simulink model "Engine_Model_HIL"  (R2016b)
settings: Solver=FixedStepDiscrete  StartTime=0.0  StopTime=inf  FixedStep=EngMdl.tiSimnTiStep_C  RelTol=1e-3  EnableMultiTasking=on
undefined symbols (not defined in the file or in its folder): EngMdl
libraries: gtlink2017rt x1, simulink x1
(part 1 of 2)
settings Model: Creator=m01wolf  LastModifiedBy=bunver
settings DataIOCC: SaveFormat=StructureWithTime  SaveOutput=off  DSMLogging=off  VisualizeSimOutput=off  SaveTime=off  StateSaveName=Results  SignalLoggingName=Results
settings OptimizationCC: BlockReduction=off  ConditionallyExecuteInputs=off  LifeSpan=inf
settings DebuggingCC: AllowSymbolicDim=off  SFUnexpectedBacktrackingDiag=warning  SFNoUnconditionalDefaultTransitionDiag=warning  SFExecutionAtInitializationDiag=none
settings ModelReferenceCC: ModelReferenceNumInstancesAllowed=Single  PropagateSignalLabelsOutOfModel=off
settings GRTTargetCC: TargetLangStandard=C89/C90 (ANSI)
settings ConfigComp: CovMetricSettings=dw  CovHtmlReporting=on  CovSaveCumulativeToWorkspaceVar=on  CovSaveSingleToWorkspaceVar=on  CovExternalEMLEnable=off

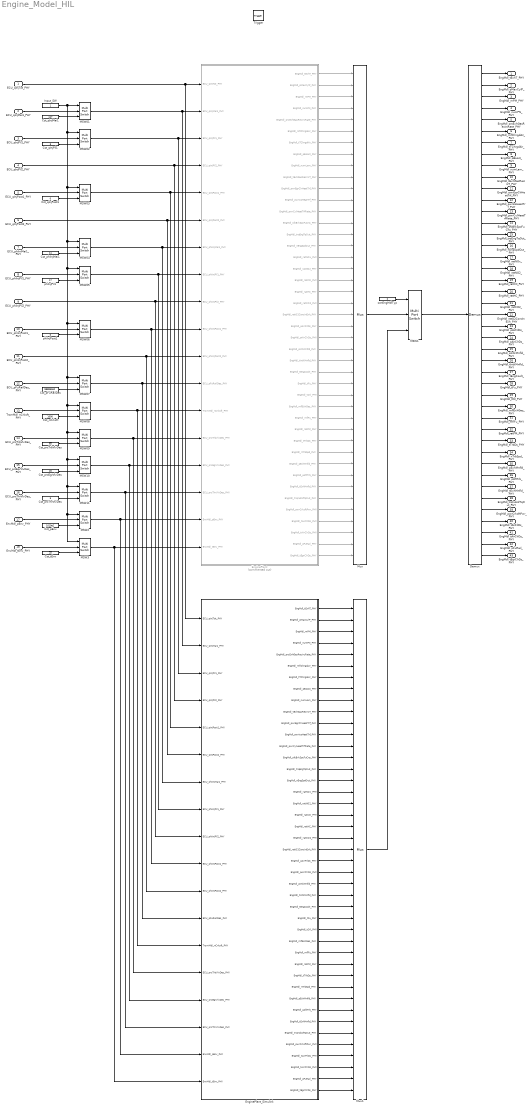
== system Engine_Model_HIL ==
  ECU_qInjTot_PHY : Inport
  ECU_qInjMai1_PHY : Inport  Port=2
  ECU_qInjPil1_PHY : Inport  Port=3
  ECU_qInjPil2_PHY : Inport  Port=4
  ECU_qInjPost1_PHY : Inport  Port=5
  ECU_qInjPost2_PHY : Inport  Port=6
  ECU_phiInjMai1_PHY : Inport  Port=7
  ECU_phiInjPil1_PHY : Inport  Port=8
  ECU_phiInjPil2_PHY : Inport  Port=9
  ECU_phiInjPost1_PHY : Inport  Port=10
  ECU_phiInjPost2_PHY : Inport  Port=11
  ECU_pFuRailDes_PHY : Inport  Port=12
  TrsmMdl_nCrksft_PHY : Inport  Port=13
  ECU_prcTrbVlvDes_PHY : Inport  Port=14
  ECU_prcEgrVlvDes_PHY : Inport  Port=15
  ECU_prcThrVlvDes_PHY : Inport  Port=16
  EnvMdl_pEnv_PHY : Inport  Port=17
  EnvMdl_tEnv_PHY : Inport  Port=18
  Trigger : TriggerPort  TriggerType=function-call  VariantControl=Variant  SampleTime=EngMdl.tiSimnTiStep_C  PortDimensions=1
  Cst_nCrksft : Constant  Value=1000  SampleTime=-1
  Cst_pEnv : Constant  Value=1010e2  SampleTime=-1
  Cst_pFuRailDes : Constant  Value=988853e2  SampleTime=-1
  Cst_phiInjMai1 : Constant  Value=11  SampleTime=-1
  Cst_prcEgrVlvDes : Constant  Value=20  SampleTime=-1
  Cst_prcThrVlvDes : Constant  Value=5  SampleTime=-1
  Cst_prcTrbVlvDes : Constant  Value=65  SampleTime=-1
  Cst_qInjMai1 : Constant  Value=147  SampleTime=-1
  Cst_qInjPil1 : Constant  Value=3  SampleTime=-1
  Cst_qInjPost1 : Constant  Value=0  SampleTime=-1
  Cst_tEnv : Constant  Value=25  SampleTime=-1
  Demux : Demux  Outputs=43
  EnginePlant : Subsystem  Commented=on
  EnginePlant_Simulink : Subsystem
  Input_SW : Constant  SampleTime=-1
  MSW01 : MultiPortSwitch  Inputs=2
  MSW02 : MultiPortSwitch  Inputs=2
  MSW03 : MultiPortSwitch  Inputs=2
  MSW04 : MultiPortSwitch  Inputs=2
  MSW05 : MultiPortSwitch  Inputs=2
  MSW06 : MultiPortSwitch  Inputs=2
  MSW07 : MultiPortSwitch  Inputs=2
  MSW08 : MultiPortSwitch  Inputs=2
  MSW09 : MultiPortSwitch  Inputs=2
  MSW{1..3,10..11} (5 alike) : MultiPortSwitch  Inputs=2
  Mux : Mux  Inputs=43
  Mux1 : Mux  Inputs=43
  phiInjPil1 : Constant  Value=17  SampleTime=-1
  phiInjPost1 : Constant  Value=0  SampleTime=-1
  swtEngMdlTyp : Constant  Value=2  SampleTime=-1
  EngMdl_tExhT_PHY : Outport  OutMin=-21  OutMax=2147
  EngMdl_pMaxCylP_PHY : Outport  Port=2  OutMin=-21  OutMax=2147
  EngMdl_mPM_PHY : Outport  Port=3  OutMin=-21  OutMax=2147
  EngMdl_numPN_PHY : Outport  Port=4  OutMin=-21  OutMax=200000000
  EngMdl_prcExhGasRecircRate_PHY : Outport  Port=5  OutMin=-21  OutMax=200
  EngMdl_mflChrgdAir_PHY : Outport  Port=6  OutMin=-21  OutMax=2147487
  EngMdl_tTChrgdAir_PHY : Outport  Port=7  OutMin=-50  OutMax=257
  EngMdl_pBoost_PHY : Outport  Port=8  OutMin=-1  OutMax=12
  EngMdl_numLam_PHY : Outport  Port=9  OutMin=-1  OutMax=15
  EngMdl_tExhGasRecircT_PHY : Outport  Port=10  OutMin=-21  OutMax=2000
  EngMdl_pwrEgrClrHeatTrf_PHY : Outport  Port=11  OutMin=-32768  OutMax=32767
  EngMdl_pwrIcoHeatTrf_PHY : Outport  Port=12  OutMin=-32768  OutMax=32767
  EngMdl_pwrCylHeatTrfRate_PHY : Outport  Port=13  OutMin=-2147483648  OutMax=2147483647
  EngMdl_sfcBrkSpcFuCns_PHY : Outport  Port=14  OutMin=-214  OutMax=2147
  EngMdl_trqEngTqOut_PHY : Outport  Port=15  OutMin=-21470  OutMax=214748
  EngMdl_nEngSpdOut_PHY : Outport  Port=16  OutMin=-21470  OutMax=21474
  EngMdl_ratNOx_PHY : Outport  Port=17  OutMin=-21  OutMax=214700
  EngMdl_ratNO2_PHY : Outport  Port=18  OutMin=-21  OutMax=214700
  EngMdl_ratCO_PHY : Outport  Port=19  OutMin=-21  OutMax=214700
  EngMdl_ratHC_PHY : Outport  Port=20  OutMin=-21  OutMax=214700
  EngMdl_ratCO2_PHY : Outport  Port=21  OutMin=-21  OutMax=20000000
  EngMdl_ratO2ConcInExh_PHY : Outport  Port=22  OutMin=-2147483648  OutMax=2147483647
  EngMdl_pAirFilDs_PHY : Outport  Port=23  OutMin=0  OutMax=1000000
  EngMdl_pAirClrDs_PHY : Outport  Port=24  OutMin=0  OutMax=1000000
  EngMdl_pIntkMnfld_PHY : Outport  Port=25  OutMin=0  OutMax=1000000
  EngMdl_tIntkMnfld_PHY : Outport  Port=26  OutMin=-250  OutMax=1000
  EngMdl_tEngCoolt_PHY : Outport  Port=27  OutMin=-250  OutMax=1000
  EngMdl_tFu_PHY : Outport  Port=28  OutMin=-250  OutMax=1000
  EngMdl_tOil_PHY : Outport  Port=29  OutMin=-250  OutMax=1000
  EngMdl_mflExhGas_PHY : Outport  Port=30
  EngMdl_mflFu_PHY : Outport  Port=31
  EngMdl_ratPM_PHY : Outport  Port=32
  EngMdl_tTrbDs_PHY : Outport  Port=33
  EngMdl_nTrbSpd_PHY : Outport  Port=34
  EngMdl_pExhMnfld_PHY : Outport  Port=35
  EngMdl_pAftTrb_PHY : Outport  Port=36
  EngMdl_tExhMnfld_PHY : Outport  Port=37
  EngMdl_trqIndcdTqOut_PHY : Outport  Port=38
  EngMdl_pwrCrksftPwr_PHY : Outport  Port=39
  EngMdl_tAirFilDs_PHY : Outport  Port=40
  EngMdl_tAirClrDs_PHY : Outport  Port=41
  EngMdl_pFuRail_PHY : Outport  Port=42
  EngMdl_tEgrClrDs_PHY : Outport  Port=43
  wires:
  ECU_qInjTot_PHY/1 -> EnginePlant_Simulink/1(ECU_qInjTot_PHY), EnginePlant/1(ECU_qInjTot_PHY)
  ECU_qInjPil2_PHY/1 -> EnginePlant/4(ECU_qInjPil2_PHY), EnginePlant_Simulink/4(ECU_qInjPil2_PHY)
  ECU_qInjPost2_PHY/1 -> EnginePlant/6(ECU_qInjPost2_PHY), EnginePlant_Simulink/6(ECU_qInjPost2_PHY)
  ECU_phiInjPil2_PHY/1 -> EnginePlant/9(ECU_phiInjPil2_PHY), EnginePlant_Simulink/9(ECU_phiInjPil2_PHY)
  ECU_phiInjPost2_PHY/1 -> EnginePlant/11(ECU_phiInjPost2_PHY), EnginePlant_Simulink/11(ECU_phiInjPost2_PHY)
  Cst_qInjMai1/1 -> MSW01/3
  Cst_qInjPil1/1 -> MSW02/3
  phiInjPil1/1 -> MSW05/3
  Cst_phiInjMai1/1 -> MSW04/3
  Cst_pFuRailDes/1 -> MSW07/3
  Cst_nCrksft/1 -> MSW08/3
  Cst_prcTrbVlvDes/1 -> MSW09/3
  Cst_prcThrVlvDes/1 -> MSW11/3
  Cst_prcEgrVlvDes/1 -> MSW10/3
  MSW01/1 -> EnginePlant/2(ECU_qInjMai1_PHY), EnginePlant_Simulink/2(ECU_qInjMai1_PHY)
  MSW02/1 -> EnginePlant/3(ECU_qInjPil1_PHY), EnginePlant_Simulink/3(ECU_qInjPil1_PHY)
  ECU_qInjPil1_PHY/1 -> MSW02/2
  ECU_qInjMai1_PHY/1 -> MSW01/2
  MSW04/1 -> EnginePlant/7(ECU_phiInjMai1_PHY), EnginePlant_Simulink/7(ECU_phiInjMai1_PHY)
  ECU_phiInjMai1_PHY/1 -> MSW04/2
  MSW05/1 -> EnginePlant/8(ECU_phiInjPil1_PHY), EnginePlant_Simulink/8(ECU_phiInjPil1_PHY)
  ECU_phiInjPil1_PHY/1 -> MSW05/2
  MSW07/1 -> EnginePlant/12(ECU_pFuRailDes_PHY), EnginePlant_Simulink/12(ECU_pFuRailDes_PHY)
  ECU_pFuRailDes_PHY/1 -> MSW07/2
  MSW08/1 -> EnginePlant/13(TrsmMdl_nCrksft_PHY), EnginePlant_Simulink/13(TrsmMdl_nCrksft_PHY)
  TrsmMdl_nCrksft_PHY/1 -> MSW08/2
  MSW09/1 -> EnginePlant/14(ECU_prcTrbVlvDes_PHY), EnginePlant_Simulink/14(ECU_prcTrbVlvDes_PHY)
  ECU_prcTrbVlvDes_PHY/1 -> MSW09/2
  ECU_prcEgrVlvDes_PHY/1 -> MSW10/2
  MSW10/1 -> EnginePlant/15(ECU_prcEgrVlvDes_PHY), EnginePlant_Simulink/15(ECU_prcEgrVlvDes_PHY)
  MSW11/1 -> EnginePlant/16(ECU_prcThrVlvDes_PHY), EnginePlant_Simulink/16(ECU_prcThrVlvDes_PHY)
  ECU_prcThrVlvDes_PHY/1 -> MSW11/2
  Input_SW/1 -> MSW02/1, MSW03/1, MSW04/1, MSW05/1, MSW06/1, MSW07/1, MSW08/1, MSW09/1, MSW10/1, MSW2/1, MSW3/1, MSW11/1, MSW01/1
  phiInjPost1/1 -> MSW06/3
  MSW06/1 -> EnginePlant/10(ECU_phiInjPost1_PHY), EnginePlant_Simulink/10(ECU_phiInjPost1_PHY)
  ECU_phiInjPost1_PHY/1 -> MSW06/2
  Cst_qInjPost1/1 -> MSW03/3
  MSW03/1 -> EnginePlant/5(ECU_qInjPost1_PHY), EnginePlant_Simulink/5(ECU_qInjPost1_PHY)
  ECU_qInjPost1_PHY/1 -> MSW03/2
  EnginePlant_Simulink/37(EngMdl_tExhMnfld_PHY) -> Mux1/37
  EnginePlant_Simulink/7(EngMdl_tTChrgdAir_PHY) -> Mux1/7
  EnginePlant_Simulink/32(EngMdl_ratPM_PHY) -> Mux1/32
  EnginePlant_Simulink/24(EngMdl_pAirClrDs_PHY) -> Mux1/24
  EnginePlant_Simulink/14(EngMdl_sfcBrkSpcFuCns_PHY) -> Mux1/14
  EnginePlant_Simulink/28(EngMdl_tFu_PHY) -> Mux1/28
  EnginePlant_Simulink/39(EngMdl_pwrCrksftPwr_PHY) -> Mux1/39
  EnginePlant_Simulink/12(EngMdl_pwrIcoHeatTrf_PHY) -> Mux1/12
  EnginePlant_Simulink/4(EngMdl_numPN_PHY) -> Mux1/4
  EnginePlant_Simulink/16(EngMdl_nEngSpdOut_PHY) -> Mux1/16
  EnginePlant_Simulink/19(EngMdl_ratCO_PHY) -> Mux1/19
  EnginePlant_Simulink/20(EngMdl_ratHC_PHY) -> Mux1/20
  EnginePlant_Simulink/21(EngMdl_ratCO2_PHY) -> Mux1/21
  EnginePlant_Simulink/6(EngMdl_mflChrgdAir_PHY) -> Mux1/6
  EnginePlant_Simulink/22(EngMdl_ratO2ConcInExh_PHY) -> Mux1/22
  EnginePlant_Simulink/27(EngMdl_tEngCoolt_PHY) -> Mux1/27
  EnginePlant_Simulink/29(EngMdl_tOil_PHY) -> Mux1/29
  EnginePlant_Simulink/36(EngMdl_pAftTrb_PHY) -> Mux1/36
  EnginePlant_Simulink/15(EngMdl_trqEngTqOut_PHY) -> Mux1/15
  EnginePlant_Simulink/38(EngMdl_trqIndcdTqOut_PHY) -> Mux1/38
  EnginePlant_Simulink/31(EngMdl_mflFu_PHY) -> Mux1/31
  EnginePlant_Simulink/11(EngMdl_pwrEgrClrHeatTrf_PHY) -> Mux1/11
  EnginePlant_Simulink/10(EngMdl_tExhGasRecircT_PHY) -> Mux1/10
  EnginePlant_Simulink/35(EngMdl_pExhMnfld_PHY) -> Mux1/35
  EnginePlant_Simulink/2(EngMdl_pMaxCylP_PHY) -> Mux1/2
  EnginePlant_Simulink/5(EngMdl_prcExhGasRecircRate_PHY) -> Mux1/5
  EnginePlant_Simulink/25(EngMdl_pIntkMnfld_PHY) -> Mux1/25
  EnginePlant_Simulink/23(EngMdl_pAirFilDs_PHY) -> Mux1/23
  EnginePlant_Simulink/13(EngMdl_pwrCylHeatTrfRate_PHY) -> Mux1/13
  EnginePlant_Simulink/26(EngMdl_tIntkMnfld_PHY) -> Mux1/26
  EnginePlant_Simulink/8(EngMdl_pBoost_PHY) -> Mux1/8
  EnginePlant_Simulink/33(EngMdl_tTrbDs_PHY) -> Mux1/33
  EnginePlant_Simulink/30(EngMdl_mflExhGas_PHY) -> Mux1/30
  EnginePlant_Simulink/1(EngMdl_tExhT_PHY) -> Mux1/1
  EnginePlant_Simulink/9(EngMdl_numLam_PHY) -> Mux1/9
  EnginePlant_Simulink/3(EngMdl_mPM_PHY) -> Mux1/3
  EnginePlant_Simulink/18(EngMdl_ratNO2_PHY) -> Mux1/18
  EnginePlant_Simulink/17(EngMdl_ratNOx_PHY) -> Mux1/17
  EnginePlant_Simulink/34(EngMdl_nTrbSpd_PHY) -> Mux1/34
  Mux/1 -> MSW1/2
  Mux1/1 -> MSW1/3
  MSW1/1 -> Demux/1
  swtEngMdlTyp/1 -> MSW1/1
  EnvMdl_pEnv_PHY/1 -> MSW2/2
  EnvMdl_tEnv_PHY/1 -> MSW3/2
  Cst_pEnv/1 -> MSW2/3
  Cst_tEnv/1 -> MSW3/3
  EnginePlant/11(EngMdl_pwrEgrClrHeatTrf_PHY) -> Mux/11
  EnginePlant/10(EngMdl_tExhGasRecircT_PHY) -> Mux/10
  EnginePlant/9(EngMdl_numLam_PHY) -> Mux/9
  EnginePlant/8(EngMdl_pBoost_PHY) -> Mux/8
  EnginePlant/7(EngMdl_tTChrgdAir_PHY) -> Mux/7
  EnginePlant/6(EngMdl_mflChrgdAir_PHY) -> Mux/6
  EnginePlant/5(EngMdl_prcExhGasRecircRate_PHY) -> Mux/5
  EnginePlant/4(EngMdl_numPN_PHY) -> Mux/4
  EnginePlant/3(EngMdl_mPM_PHY) -> Mux/3
  EnginePlant/2(EngMdl_pMaxCylP_PHY) -> Mux/2
  EnginePlant/1(EngMdl_tExhT_PHY) -> Mux/1
  EnginePlant/43(EngMdl_tEgrClrDs_PHY) -> Mux/43
  EnginePlant/42(EngMdl_pFuRail_PHY) -> Mux/42
  EnginePlant/41(EngMdl_tAirClrDs_PHY) -> Mux/41
  EnginePlant/40(EngMdl_tAirFilDs_PHY) -> Mux/40
  EnginePlant/39(EngMdl_pwrCrksftPwr_PHY) -> Mux/39
  EnginePlant/38(EngMdl_trqIndcdTqOut_PHY) -> Mux/38
  EnginePlant/37(EngMdl_tExhMnfld_PHY) -> Mux/37
  EnginePlant/36(EngMdl_pAftTrb_PHY) -> Mux/36
  EnginePlant/35(EngMdl_pExhMnfld_PHY) -> Mux/35
  EnginePlant/34(EngMdl_nTrbSpd_PHY) -> Mux/34
  EnginePlant/33(EngMdl_tTrbDs_PHY) -> Mux/33
  EnginePlant/32(EngMdl_ratPM_PHY) -> Mux/32
  EnginePlant/31(EngMdl_mflFu_PHY) -> Mux/31
  EnginePlant/30(EngMdl_mflExhGas_PHY) -> Mux/30
  EnginePlant/29(EngMdl_tOil_PHY) -> Mux/29
  EnginePlant/28(EngMdl_tFu_PHY) -> Mux/28
  EnginePlant/27(EngMdl_tEngCoolt_PHY) -> Mux/27
  EnginePlant/26(EngMdl_tIntkMnfld_PHY) -> Mux/26
  EnginePlant/25(EngMdl_pIntkMnfld_PHY) -> Mux/25
  EnginePlant/24(EngMdl_pAirClrDs_PHY) -> Mux/24
  EnginePlant/23(EngMdl_pAirFilDs_PHY) -> Mux/23
  EnginePlant/22(EngMdl_ratO2ConcInExh_PHY) -> Mux/22
  EnginePlant/21(EngMdl_ratCO2_PHY) -> Mux/21
  EnginePlant/20(EngMdl_ratHC_PHY) -> Mux/20
  EnginePlant/19(EngMdl_ratCO_PHY) -> Mux/19
  EnginePlant/18(EngMdl_ratNO2_PHY) -> Mux/18
  EnginePlant/17(EngMdl_ratNOx_PHY) -> Mux/17
  EnginePlant/16(EngMdl_nEngSpdOut_PHY) -> Mux/16
  EnginePlant/15(EngMdl_trqEngTqOut_PHY) -> Mux/15
  EnginePlant/14(EngMdl_sfcBrkSpcFuCns_PHY) -> Mux/14
  EnginePlant/13(EngMdl_pwrCylHeatTrfRate_PHY) -> Mux/13
  EnginePlant/12(EngMdl_pwrIcoHeatTrf_PHY) -> Mux/12
  MSW2/1 -> EnginePlant_Simulink/17(EnvMdl_pEnv_PHY), EnginePlant/17(EnvMdl_pEnv_PHY)
  MSW3/1 -> EnginePlant_Simulink/18(EnvMdl_tEnv_PHY), EnginePlant/18(EnvMdl_tEnv_PHY)
  Demux/42 -> EngMdl_pFuRail_PHY/1
  Demux/41 -> EngMdl_tAirClrDs_PHY/1
  Demux/43 -> EngMdl_tEgrClrDs_PHY/1
  Demux/40 -> EngMdl_tAirFilDs_PHY/1
  Demux/9 -> EngMdl_numLam_PHY/1
  Demux/10 -> EngMdl_tExhGasRecircT_PHY/1
  Demux/11 -> EngMdl_pwrEgrClrHeatTrf_PHY/1
  Demux/12 -> EngMdl_pwrIcoHeatTrf_PHY/1
  Demux/13 -> EngMdl_pwrCylHeatTrfRate_PHY/1
  Demux/14 -> EngMdl_sfcBrkSpcFuCns_PHY/1
  Demux/1 -> EngMdl_tExhT_PHY/1
  Demux/2 -> EngMdl_pMaxCylP_PHY/1
  Demux/3 -> EngMdl_mPM_PHY/1
  Demux/21 -> EngMdl_ratCO2_PHY/1
  Demux/22 -> EngMdl_ratO2ConcInExh_PHY/1
  Demux/23 -> EngMdl_pAirFilDs_PHY/1
  Demux/24 -> EngMdl_pAirClrDs_PHY/1
  Demux/25 -> EngMdl_pIntkMnfld_PHY/1
  Demux/26 -> EngMdl_tIntkMnfld_PHY/1
  Demux/15 -> EngMdl_trqEngTqOut_PHY/1
  Demux/16 -> EngMdl_nEngSpdOut_PHY/1
  Demux/17 -> EngMdl_ratNOx_PHY/1
  Demux/18 -> EngMdl_ratNO2_PHY/1
  Demux/19 -> EngMdl_ratCO_PHY/1
  Demux/20 -> EngMdl_ratHC_PHY/1
  Demux/4 -> EngMdl_numPN_PHY/1
  Demux/5 -> EngMdl_prcExhGasRecircRate_PHY/1
  Demux/6 -> EngMdl_mflChrgdAir_PHY/1
  Demux/7 -> EngMdl_tTChrgdAir_PHY/1
  Demux/8 -> EngMdl_pBoost_PHY/1
  Demux/27 -> EngMdl_tEngCoolt_PHY/1
  Demux/28 -> EngMdl_tFu_PHY/1
  Demux/29 -> EngMdl_tOil_PHY/1
  Demux/30 -> EngMdl_mflExhGas_PHY/1
  Demux/31 -> EngMdl_mflFu_PHY/1
  Demux/32 -> EngMdl_ratPM_PHY/1
  Demux/33 -> EngMdl_tTrbDs_PHY/1
  Demux/34 -> EngMdl_nTrbSpd_PHY/1
  Demux/35 -> EngMdl_pExhMnfld_PHY/1
  Demux/36 -> EngMdl_pAftTrb_PHY/1
  Demux/37 -> EngMdl_tExhMnfld_PHY/1
  Demux/38 -> EngMdl_trqIndcdTqOut_PHY/1
  Demux/39 -> EngMdl_pwrCrksftPwr_PHY/1
  EnginePlant_Simulink/40(EngMdl_tAirFilDs_PHY) -> Mux1/40
  EnginePlant_Simulink/41(EngMdl_tAirClrDs_PHY) -> Mux1/41
  EnginePlant_Simulink/42(EngMdl_pFuRail_PHY) -> Mux1/42
  EnginePlant_Simulink/43(EngMdl_tEgrClrDs_PHY) -> Mux1/43

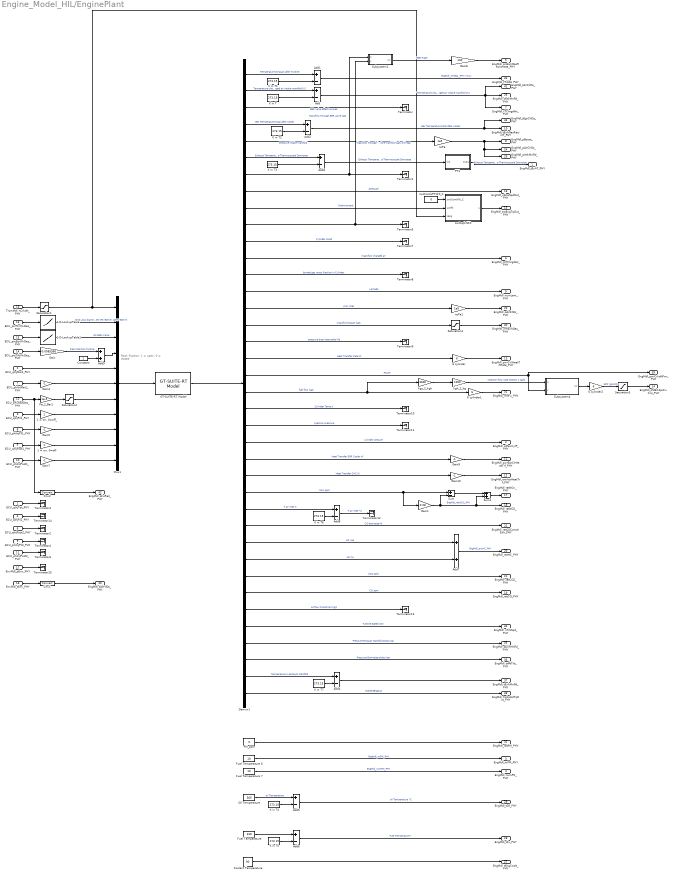
== system Engine_Model_HIL/EnginePlant ==
  note: Rack Position: 1 = open,
      | 			  0 = closed
  ECU_qInjTot_PHY : Inport
  ECU_qInjMai1_PHY : Inport  Port=2
  ECU_qInjPil1_PHY : Inport  Port=3
  ECU_qInjPil2_PHY : Inport  Port=4
  ECU_qInjPost1_PHY : Inport  Port=5
  ECU_qInjPost2_PHY : Inport  Port=6
  ECU_phiInjMai1_PHY : Inport  Port=7
  ECU_phiInjPil1_PHY : Inport  Port=8
  ECU_phiInjPil2_PHY : Inport  Port=9
  ECU_phiInjPost1_PHY : Inport  Port=10
  ECU_phiInjPost2_PHY : Inport  Port=11
  ECU_pFuRailDes_PHY : Inport  Port=12
  TrsmMdl_nCrksft_PHY : Inport  Port=13
  ECU_prcTrbVlvDes_PHY : Inport  Port=14
  ECU_prcEgrVlvDes_PHY : Inport  Port=15
  ECU_prcThrVlvDes_PHY : Inport  Port=16
  EnvMdl_pEnv_PHY : Inport  Port=17
  EnvMdl_tEnv_PHY : Inport  Port=18
  "1 = on, 0=off" : Gain
  "1 = on, 0=off_" : Gain
  1-D LookupTable : Lookup_n-D  NumberOfTableDimensions=1  BreakpointsForDimension1=[5 100]  Table=[80 0]  ExtrapMethod=Clip  UseLastTableValue=on  InternalRulePriority=Speed  RndMeth=Simplest  InputSameDT=on
  1-D LookupTable1 : Lookup_n-D  NumberOfTableDimensions=1  BreakpointsForDimension1=[0 100]  Table=[0 90]  ExtrapMethod=Clip  UseLastTableValue=on  InternalRulePriority=Speed  RndMeth=Simplest  InputSameDT=on
  6 cylinder : Gain  Gain=6
  6 cylinder1 : Gain  Gain=6
  6 cylinder2 : Gain  Gain=6
  Add{,1..6,8} (8 alike) : Sum  Inputs=+-
  Add7 : Sum
  Add9 : Sum
  Cnv1 : DataTypeConversion
  Cnv2 : DataTypeConversion
  Constant : Constant
  Coolant Temperature : Constant  Value=90
  Demux1 : Demux  Outputs=38
  "Fuel Temperature " : Constant  Value=330
  Fuel Temperature 6 : Constant  Value=10
  Fuel Temperature 7 : Constant  Value=10
  GT-SUITE-RT Model : gtlink2017rt/GT-SUITE-RT Model  gti_fname=OptiTruck_RT_enginemodel_v0  gti_dur=SIMULINK  gti_msg=No runtime messages  gti_dt=EngMdl.tiSimnTiStep_C  gti_ni=11  gti_no=38  gti_parnam='ign'  gti_parval='ign'  gti_cylnam='ign'  gti_nrtpr=-1
      settings: AttributesFormatString=(%<gti_fname>.dat)
  Gain : Gain  Gain=-0.0085366
  Gain1 : Gain  Gain=0.08
  Gain{4..5,7,9..10} (5 alike) : Gain  Gain=-1
  Gain8 : Gain  Gain=100
  K in T{,1..7} (8 alike) : Constant  Value=273.15
  Mux1 : Mux  Inputs=11
  Oil Temperature : Constant  Value=365
  PM_ppm : Constant  Value=0
  PT1 : Subsystem
  Pa_2_Bar1 : Gain  Gain=1e-5
  Saturation1 : Saturate  UpperLimit=2500  LowerLimit=0
  Saturation2 : Saturate  UpperLimit=2500  LowerLimit=0
  Saturation3 : Saturate  UpperLimit=800  LowerLimit=0
  Saturation4 : Saturate  UpperLimit=inf  LowerLimit=1/3600
  Subsystem1 : Subsystem  mask(DivideByZeroProtectionPositive){MinimumDenominator=1.0}
      mask prompts: MinimumDenominator "Minimum value of denominator"
      mask help: This block behaves similar to the Simulink divide block, except that it prevents crashing during simulation when Y becomes 0.
      settings: AttributesFormatString=<YMin=%<MinimumDenominator>>
      mask Display:
      | disp('Zero Div\nPositive')
      | port_label('input', 1, 'X')
      | port_label('input', 2, 'Y')
      | port_label('output', 1, 'X/Y')
  Subsystem4 : Subsystem  mask(DivideByZeroProtectionPositive){MinimumDenominator=1.0}
      mask prompts: MinimumDenominator "Minimum value of denominator"
      mask help: This block behaves similar to the Simulink divide block, except that it prevents crashing during simulation when Y becomes 0.
      settings: AttributesFormatString=<YMin=%<MinimumDenominator>>
      mask Display:
      | disp('Zero Div\nPositive')
      | port_label('input', 1, 'X')
      | port_label('input', 2, 'Y')
      | port_label('output', 1, 'X/Y')
  Sum : Sum  Inputs=+-
  Sum1 : Sum
  Terminator{,1..15} (16 alike) : Terminator
  kgh_2_hg : Gain  Gain=1000
  kgs_2_kgh : Gain  Gain=3600
  swtCombPT1Flt_C : Constant  Value=0  SampleTime=-1
  swttrqCrSFlt : Subsystem
  toPa : Gain  Gain=1e5
  toPa1 : Gain  Gain=1e5
  EngMdl_tExhT_PHY : Outport
  EngMdl_pMaxCylP_PHY : Outport  Port=2
  EngMdl_mPM_PHY : Outport  Port=3
  EngMdl_numPN_PHY : Outport  Port=4
  EngMdl_prcExhGasRecircRate_PHY : Outport  Port=5
  EngMdl_mflChrgdAir_PHY : Outport  Port=6
  EngMdl_tTChrgdAir_PHY : Outport  Port=7
  EngMdl_pBoost_PHY : Outport  Port=8
  EngMdl_numLam_PHY : Outport  Port=9
  EngMdl_tExhGasRecircT_PHY : Outport  Port=10
  EngMdl_pwrEgrClrHeatTrf_PHY : Outport  Port=11
  EngMdl_pwrIcoHeatTrf_PHY : Outport  Port=12
  EngMdl_pwrCylHeatTrfRate_PHY : Outport  Port=13
  EngMdl_sfcBrkSpcFuCns_PHY : Outport  Port=14
  EngMdl_trqEngTqOut_PHY : Outport  Port=15
  EngMdl_nEngSpdOut_PHY : Outport  Port=16
  EngMdl_ratNOx_PHY : Outport  Port=17
  EngMdl_ratNO2_PHY : Outport  Port=18
  EngMdl_ratCO_PHY : Outport  Port=19
  EngMdl_ratHC_PHY : Outport  Port=20
  EngMdl_ratCO2_PHY : Outport  Port=21
  EngMdl_ratO2ConcInExh_PHY : Outport  Port=22
  EngMdl_pAirFilDs_PHY : Outport  Port=23
  EngMdl_pAirClrDs_PHY : Outport  Port=24
  EngMdl_pIntkMnfld_PHY : Outport  Port=25
  EngMdl_tIntkMnfld_PHY : Outport  Port=26
  EngMdl_tEngCoolt_PHY : Outport  Port=27
  EngMdl_tFu_PHY : Outport  Port=28
  EngMdl_tOil_PHY : Outport  Port=29
  EngMdl_mflExhGas_PHY : Outport  Port=30
  EngMdl_mflFu_PHY : Outport  Port=31
  EngMdl_ratPM_PHY : Outport  Port=32
  EngMdl_tTrbDs_PHY : Outport  Port=33
  EngMdl_nTrbSpd_PHY : Outport  Port=34
  EngMdl_pExhMnfld_PHY : Outport  Port=35
  EngMdl_pAftTrb_PHY : Outport  Port=36
  EngMdl_tExhMnfld_PHY : Outport  Port=37
  EngMdl_trqIndcdTqOut_PHY : Outport  Port=38
  EngMdl_pwrCrksftPwr_PHY : Outport  Port=39
  EngMdl_tAirFilDs_PHY : Outport  Port=40
  EngMdl_tAirClrDs_PHY : Outport  Port=41
  EngMdl_pFuRail_PHY : Outport  Port=42
  EngMdl_tEgrClrDs_PHY : Outport  Port=43
  wires:
  ECU_qInjPil2_PHY/1 -> Terminator14/1
  1-D LookupTable/1 -> Mux1/2  "Grid Loss diameter 0%-80mm 100%-80mm"
  Gain/1 -> Add9/1  "Rack Position Turbine"
  toPa1/1 -> EngMdl_pAirFilDs_PHY/1
  Mux1/1 -> GT-SUITE-RT Model/1
  ECU_qInjTot_PHY/1 -> Terminator3/1
  ECU_phiInjPost2_PHY/1 -> Terminator6/1
  Saturation1/1 -> swttrqCrSFlt/3(nEng), Mux1/1
  1-D LookupTable1/1 -> Mux1/3  "phi EGR-Valve"
  Gain5/1 -> Mux1/9
  Gain4/1 -> Mux1/6
  "1 = on, 0=off_"/1 -> Mux1/8
  Pa_2_Bar1/1 -> Saturation2/1
  ECU_phiInjPost1_PHY/1 -> Gain7/1
  ECU_phiInjPil2_PHY/1 -> Terminator4/1
  ECU_qInjPost2_PHY/1 -> Terminator2/1
  Coolant Temperature/1 -> EngMdl_tEngCoolt_PHY/1
  Add6/1 -> EngMdl_tFu_PHY/1  "Fuel Temperature °"
  Oil Temperature/1 -> Add5/1  "oil Temperature"
  K in T5/1 -> Add6/2
  Gain1/1 -> Sum/2, Sum1/2, EngMdl_ratNO2_PHY/1  "EngMdl_ratNO2_PHY"
  Add7/1 -> EngMdl_ratHC_PHY/1  "EngMdl_prcHC_PHY"
  Fuel Temperature 6/1 -> EngMdl_mPM_PHY/1  "EngMdl_mPM_PHY"
  Add5/1 -> EngMdl_tOil_PHY/1  "oil Temperature °C"
  K in T4/1 -> Add5/2
  Fuel Temperature 7/1 -> EngMdl_numPN_PHY/1  "EngMdl_numPN_PHY"
  "Fuel Temperature "/1 -> Add6/1
  Saturation2/1 -> Mux1/7
  swtCombPT1Flt_C/1 -> swttrqCrSFlt/1(swtCombFlt_C)
  swttrqCrSFlt/1(u) -> EngMdl_trqEngTqOut_PHY/1
  TrsmMdl_nCrksft_PHY/1 -> Saturation1/1
  ECU_prcEgrVlvDes_PHY/1 -> 1-D LookupTable1/1
  ECU_prcTrbVlvDes_PHY/1 -> Gain/1
  ECU_prcThrVlvDes_PHY/1 -> 1-D LookupTable/1
  ECU_qInjMai1_PHY/1 -> Mux1/5
  ECU_phiInjMai1_PHY/1 -> Gain4/1
  ECU_pFuRailDes_PHY/1 -> Cnv2/1, Pa_2_Bar1/1
  ECU_qInjPil1_PHY/1 -> "1 = on, 0=off_"/1
  ECU_phiInjPil1_PHY/1 -> Gain5/1
  PM_ppm/1 -> EngMdl_ratPM_PHY/1
  Demux1/13 -> Terminator8/1  "burned gas mass fraction in Cylinder"
  Demux1/5 -> toPa/1  "pressure intake manifold"
  Demux1/2 -> Add/1  "Temperature charged air intake manifold [K]"
  K in T/1 -> Add/2
  Demux1/16 -> Saturation4/1  "massflo exhaust kg/s"
  Add/1 -> EngMdl_tAirClrDs_PHY/1, EngMdl_tTChrgdAir_PHY/1, EngMdl_tIntkMnfld_PHY/1  "Temperature charged air intake manifold [K]"
  K in T1/1 -> Add1/2
  Demux1/7 -> Terminator1/1, Subsystem1/1(X)  "Massflow through EGR valve kg/s"
  Demux1/8 -> EngMdl_nEngSpdOut_PHY/1  "Drehzahl"
  Demux1/17 -> Terminator9/1  "pressure drop intercooler Pa"
  K in T6/1 -> Add8/2
  K in T3/1 -> Add3/2
  K in T2/1 -> Add2/2
  Add2/1 -> EngMdl_tEgrClrDs_PHY/1, EngMdl_tExhGasRecircT_PHY/1  "EGr Temperature total after cooler"
  Demux1/18 -> 6 cylinder/1  "Heat Transfer Rate W"
  Demux1/9 -> swttrqCrSFlt/2(uUnflt)  "Drehmoment"
  Demux1/32 -> EngMdl_ratCO_PHY/1  "CO ppm"
  Demux1/34 -> EngMdl_nTrbSpd_PHY/1  "Turbine Speed rpm"
  Demux1/22 -> Terminator11/1  "injection pressure"
  Add1/1 -> EngMdl_tTrbDs_PHY/1  "EngMdl_tTrbDs_PHY [°C]>"
  Demux1/12 -> EngMdl_mflChrgdAir_PHY/1  "massflow charged air"
  Demux1/14 -> EngMdl_numLam_PHY/1  "Lambda"
  Demux1/20 -> kgs_2_kgh/1, 6 cylinder1/1  "fuel flow kg/s"
  Demux1/1 -> Add1/1  "Temperature exhaust after Turbine"
  Demux1/6 -> Add3/1  "Exhaust Temperature Thermocouple Downpipe"
  Demux1/15 -> toPa1/1  "p air inlet"
  Demux1/4 -> Add2/1  "EGr Temperature total after cooler"
  Demux1/23 -> EngMdl_pMaxCylP_PHY/1  "cylinder presure"
  Demux1/29 -> Add7/1  "HC vap"
  Demux1/27 -> Add8/1  "T air inlet K"
  Demux1/33 -> Terminator13/1  "Airflow Cranktrain kg/h"
  Demux1/25 -> Gain10/1  "Heat Transfer CAC W"
  Demux1/3 -> Terminator/1  "EGR valve effective area"
  Demux1/24 -> Gain9/1  "Heat Transfer EGR Cooler W"
  Demux1/31 -> EngMdl_ratCO2_PHY/1  "CO2 ppm"
  Demux1/26 -> Gain1/1, Sum/1  "NOx ppm"
  Demux1/10 -> Subsystem1/2(Y), Terminator5/1  "Massflow through \"grid loss\" before manifold kg/s with egr"
  Demux1/30 -> Add7/2  "HC liq"
  Add3/1 -> PT1/1(In1)  "Exhaust Temperature Thermocouple Downpipe"
  GT-SUITE-RT Model/1 -> Demux1/1
  Subsystem1/1(XY) -> Gain8/1  "EGR-Rate"
  Demux1/28 -> EngMdl_ratO2ConcInExh_PHY/1  "O2 downpipe %"
  Demux1/11 -> Terminator7/1  "Cylinder HV50"
  toPa/1 -> EngMdl_pAirClrDs_PHY/1, EngMdl_pIntkMnfld_PHY/1, EngMdl_pBoost_PHY/1
  6 cylinder2/1 -> Saturation3/1  "bsfc [g/kWh]"
  Demux1/19 -> EngMdl_pwrCrksftPwr_PHY/1, Subsystem4/2(Y)  "Power"
  kgs_2_kgh/1 -> kgh_2_hg/1
  kgh_2_hg/1 -> Subsystem4/1(X)  "injection flow rate Injector 1 [g/h]"
  Demux1/21 -> Terminator10/1  "Cylinder Temp K"
  Subsystem4/1(XY) -> 6 cylinder2/1
  Add9/1 -> Mux1/4
  Constant/1 -> Add9/2
  ECU_qInjPost1_PHY/1 -> "1 = on, 0=off"/1
  Gain7/1 -> Mux1/11
  "1 = on, 0=off"/1 -> Mux1/10
  Demux1/35 -> EngMdl_pExhMnfld_PHY/1  "Pressure Exhaust Manifold static bar"
  Demux1/36 -> EngMdl_pAftTrb_PHY/1  "Pressure Downpipe static bar"
  Gain8/1 -> EngMdl_prcExhGasRecircRate_PHY/1
  Saturation3/1 -> EngMdl_sfcBrkSpcFuCns_PHY/1
  Add8/1 -> Terminator12/1  "T air inlet °C"
  Gain9/1 -> EngMdl_pwrEgrClrHeatTrf_PHY/1
  Gain10/1 -> EngMdl_pwrIcoHeatTrf_PHY/1
  6 cylinder/1 -> EngMdl_pwrCylHeatTrfRate_PHY/1
  PT1/1(Out1) -> EngMdl_tExhT_PHY/1  "Exhaust Temperature Thermocouple Downpipe"
  Demux1/38 -> EngMdl_trqIndcdTqOut_PHY/1  "IndcdTqEngOut"
  Sum/1 -> Sum1/1
  Sum1/1 -> EngMdl_ratNOx_PHY/1
  Saturation4/1 -> EngMdl_mflExhGas_PHY/1
  Demux1/37 -> Add4/1  "Temperature in Exhaust Manifold"
  Add4/1 -> EngMdl_tExhMnfld_PHY/1
  K in T7/1 -> Add4/2
  6 cylinder1/1 -> EngMdl_mflFu_PHY/1
  Cnv1/1 -> EngMdl_tAirFilDs_PHY/1
  EnvMdl_tEnv_PHY/1 -> Cnv1/1
  EnvMdl_pEnv_PHY/1 -> Terminator15/1
  Cnv2/1 -> EngMdl_pFuRail_PHY/1

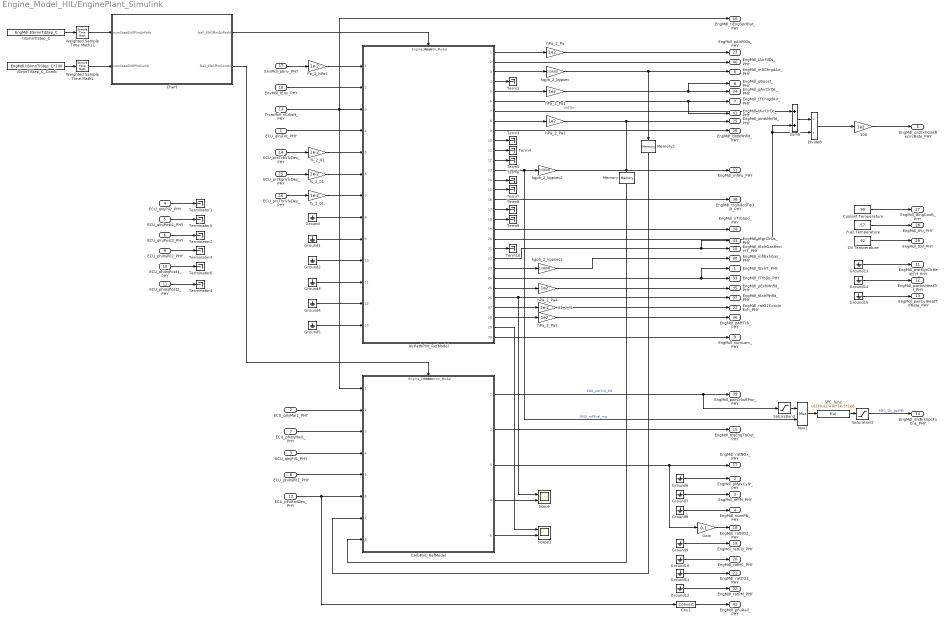
== system Engine_Model_HIL/EnginePlant_Simulink ==
  ECU_qInjTot_PHY : Inport
  ECU_qInjMai1_PHY : Inport  Port=2
  ECU_qInjPil1_PHY : Inport  Port=3
  ECU_qInjPil2_PHY : Inport  Port=4
  ECU_qInjPost1_PHY : Inport  Port=5
  ECU_qInjPost2_PHY : Inport  Port=6
  ECU_phiInjMai1_PHY : Inport  Port=7
  ECU_phiInjPil1_PHY : Inport  Port=8
  ECU_phiInjPil2_PHY : Inport  Port=9
  ECU_phiInjPost1_PHY : Inport  Port=10
  ECU_phiInjPost2_PHY : Inport  Port=11
  ECU_pFuRailDes_PHY : Inport  Port=12
  TrsmMdl_nCrksft_PHY : Inport  Port=13
  ECU_prcTrbVlvDes_PHY : Inport  Port=14
  ECU_prcEgrVlvDes_PHY : Inport  Port=15
  ECU_prcThrVlvDes_PHY : Inport  Port=16
  EnvMdl_pEnv_PHY : Inport  Port=17
  EnvMdl_tEnv_PHY : Inport  Port=18
  %_2_01 : Gain  Gain=1e-2
  %_2_01, : Gain  Gain=1e-2
  %_2_01. : Gain  Gain=1e-2
  01_2_% : Gain  Gain=1e-2
  100 : Gain  Gain=1e2
  AirPathPlnt_RefModel : ModelReference  ModelNameDialog=Engine_Airpath_Model.slx  ModelReferenceVersion=1.253  TriggerPortName=Trigger  TriggerPortTriggerType=function-call  TriggerPortStatesWhenEnabling=held
  Chart : Stateflow chart
  CmbPlnt_RefModel : ModelReference  ModelNameDialog=Engine_Combustion_Model.slx  ModelReferenceVersion=1.251  TriggerPortName=Trigger  TriggerPortTriggerType=function-call  TriggerPortStatesWhenEnabling=held
  Cnv1 : DataTypeConversion
  Coolant Temperature : Constant  Value=90
  Divide8 : Product  Inputs=*/
  "Fuel Temperature " : Constant  Value=57
  Gain : Gain  Gain=0.1
  Ground{,1..15} (16 alike) : Ground
  Memory : Memory  X0=1100e2  InheritSampleTime=on
  Memory1 : Memory  InheritSampleTime=on
  Mux1 : Mux  Inputs=2
  Oil Temperature : Constant  Value=92
  Pa_2_hPa1 : Gain  Gain=1e-2
  SFC_func : Fcn  Expr=u(2)/(u(1)+0)*1e-3*1e6
  Saturation2 : Saturate  UpperLimit=500  LowerLimit=0
  Saturation3 : Saturate  UpperLimit=inf  LowerLimit=1e-3
  Scope : Scope  NumInputPorts=2
  Scope1 : Scope  NumInputPorts=2
  Sum5 : Sum
  Term{2..10} (9 alike) : Terminator
  Terminator{1..6} (6 alike) : Terminator
  Weighted Sample Time Math1 : SampleTimeMath  TsampMathOp=/  OutDataTypeStr=Inherit: Inherit via back propagation  RndMeth=Round
  Weighted Sample Time Math11 : SampleTimeMath  TsampMathOp=/  OutDataTypeStr=Inherit: Inherit via back propagation  RndMeth=Round
  hPa_2_Pa{,1..2,4..5} (5 alike) : Gain  Gain=1e2
  iSimnTiStep_C_Comb : Constant  Value=EngMdl.tiSimnTiStep_C*100  SampleTime=-1
  kgph_2_kgpsec : Gain  Gain=1/3600
  kgph_2_kgpsec1 : Gain  Gain=1/3600
  kgph_2_kgpsec2 : Gain  Gain=1/3600
  tiSimnTiStep_C : Constant  Value=EngMdl.tiSimnTiStep_C  SampleTime=-1
  EngMdl_tExhT_PHY : Outport
  EngMdl_pMaxCylP_PHY : Outport  Port=2
  EngMdl_mPM_PHY : Outport  Port=3
  EngMdl_numPN_PHY : Outport  Port=4
  EngMdl_prcExhGasRecircRate_PHY : Outport  Port=5
  EngMdl_mflChrgdAir_PHY : Outport  Port=6
  EngMdl_tTChrgdAir_PHY : Outport  Port=7
  EngMdl_pBoost_PHY : Outport  Port=8
  EngMdl_numLam_PHY : Outport  Port=9
  EngMdl_tExhGasRecircT_PHY : Outport  Port=10
  EngMdl_pwrEgrClrHeatTrf_PHY : Outport  Port=11
  EngMdl_pwrIcoHeatTrf_PHY : Outport  Port=12
  EngMdl_pwrCylHeatTrfRate_PHY : Outport  Port=13
  EngMdl_sfcBrkSpcFuCns_PHY : Outport  Port=14
  EngMdl_trqEngTqOut_PHY : Outport  Port=15
  EngMdl_nEngSpdOut_PHY : Outport  Port=16
  EngMdl_ratNOx_PHY : Outport  Port=17
  EngMdl_ratNO2_PHY : Outport  Port=18
  EngMdl_ratCO_PHY : Outport  Port=19
  EngMdl_ratHC_PHY : Outport  Port=20
  EngMdl_ratCO2_PHY : Outport  Port=21
  EngMdl_ratO2ConcInExh_PHY : Outport  Port=22
  EngMdl_pAirFilDs_PHY : Outport  Port=23
  EngMdl_pAirClrDs_PHY : Outport  Port=24
  EngMdl_pIntkMnfld_PHY : Outport  Port=25
  EngMdl_tIntkMnfld_PHY : Outport  Port=26
  EngMdl_tEngCoolt_PHY : Outport  Port=27
  EngMdl_tFu_PHY : Outport  Port=28
  EngMdl_tOil_PHY : Outport  Port=29
  EngMdl_mflExhGas_PHY : Outport  Port=30
  EngMdl_mflFu_PHY : Outport  Port=31
  EngMdl_ratPM_PHY : Outport  Port=32
  EngMdl_tTrbDs_PHY : Outport  Port=33
  EngMdl_nTrbSpd_PHY : Outport  Port=34
  EngMdl_pExhMnfld_PHY : Outport  Port=35
  EngMdl_pAftTrb_PHY : Outport  Port=36
  EngMdl_tExhMnfld_PHY : Outport  Port=37
  EngMdl_trqIndcdTqOut_PHY : Outport  Port=38
  EngMdl_pwrCrksftPwr_PHY : Outport  Port=39
  EngMdl_tAirFilDs_PHY : Outport  Port=40
  EngMdl_tAirClrDs_PHY : Outport  Port=41
  EngMdl_pFuRail_PHY : Outport  Port=42
  EngMdl_tEgrClrDs_PHY : Outport  Port=43
  wires:
  ECU_qInjPost1_PHY/1 -> Terminator5/1
  ECU_phiInjPil1_PHY/1 -> CmbPlnt_RefModel/5
  ECU_qInjPil1_PHY/1 -> CmbPlnt_RefModel/4
  ECU_pFuRailDes_PHY/1 -> Cnv1/1, CmbPlnt_RefModel/6
  ECU_phiInjMai1_PHY/1 -> CmbPlnt_RefModel/3
  ECU_prcThrVlvDes_PHY/1 -> %_2_01,/1
  ECU_prcTrbVlvDes_PHY/1 -> %_2_01/1
  ECU_prcEgrVlvDes_PHY/1 -> %_2_01./1
  ECU_qInjPost2_PHY/1 -> Terminator2/1
  ECU_phiInjPil2_PHY/1 -> Terminator3/1
  ECU_phiInjPost1_PHY/1 -> Terminator6/1
  ECU_phiInjPost2_PHY/1 -> Terminator4/1
  ECU_qInjPil2_PHY/1 -> Terminator1/1
  Coolant Temperature/1 -> EngMdl_tEngCoolt_PHY/1
  01_2_%/1 -> EngMdl_ratO2ConcInExh_PHY/1
  Oil Temperature/1 -> EngMdl_tOil_PHY/1
  TrsmMdl_nCrksft_PHY/1 -> EngMdl_nEngSpdOut_PHY/1, CmbPlnt_RefModel/1, AirPathPlnt_RefModel/3
  Ground15/1 -> EngMdl_pwrCylHeatTrfRate_PHY/1
  AirPathPlnt_RefModel/9 -> EngMdl_tIntkMnfld_PHY/1
  Ground6/1 -> EngMdl_pMaxCylP_PHY/1
  AirPathPlnt_RefModel/30 -> EngMdl_numLam_PHY/1
  Ground7/1 -> EngMdl_mPM_PHY/1
  kgph_2_kgpsec/1 -> EngMdl_mflChrgdAir_PHY/1, Memory1/1
  AirPathPlnt_RefModel/22 -> EngMdl_tEgrClrDs_PHY/1, EngMdl_tExhGasRecircT_PHY/1
  hPa_2_Pa2/1 -> Memory/1, EngMdl_pIntkMnfld_PHY/1
  Ground9/1 -> EngMdl_ratCO_PHY/1
  Ground10/1 -> EngMdl_ratHC_PHY/1
  hPa_2_Pa1/1 -> EngMdl_pBoost_PHY/1, EngMdl_pAirClrDs_PHY/1
  "Fuel Temperature "/1 -> EngMdl_tFu_PHY/1
  Ground14/1 -> EngMdl_pwrIcoHeatTrf_PHY/1
  Ground8/1 -> EngMdl_numPN_PHY/1
  hPa_2_Pa/1 -> EngMdl_pAirFilDs_PHY/1
  100/1 -> EngMdl_prcExhGasRecircRate_PHY/1
  Ground11/1 -> EngMdl_ratCO2_PHY/1
  Ground13/1 -> EngMdl_pwrEgrClrHeatTrf_PHY/1
  AirPathPlnt_RefModel/23 -> kgph_2_kgpsec1/1
  Ground12/1 -> EngMdl_ratPM_PHY/1
  AirPathPlnt_RefModel/26 -> Scope/1, EngMdl_tExhMnfld_PHY/1
  AirPathPlnt_RefModel/19 -> EngMdl_nTrbSpd_PHY/1
  hPa_2_Pa4/1 -> EngMdl_pExhMnfld_PHY/1
  hPa_2_Pa5/1 -> EngMdl_pAftTrb_PHY/1
  AirPathPlnt_RefModel/16 -> EngMdl_trqIndcdTqOut_PHY/1
  Chart/1(fcall_ENGPlntAirPath()) -> AirPathPlnt_RefModel/Trigger
  EnvMdl_pEnv_PHY/1 -> Pa_2_hPa1/1
  ECU_qInjMai1_PHY/1 -> CmbPlnt_RefModel/2
  Pa_2_hPa1/1 -> AirPathPlnt_RefModel/1
  Ground5/1 -> AirPathPlnt_RefModel/13
  %_2_01/1 -> AirPathPlnt_RefModel/5
  %_2_01./1 -> AirPathPlnt_RefModel/6
  %_2_01,/1 -> AirPathPlnt_RefModel/7
  Ground4/1 -> AirPathPlnt_RefModel/12
  Ground3/1 -> AirPathPlnt_RefModel/11
  Ground2/1 -> AirPathPlnt_RefModel/10
  Ground/1 -> AirPathPlnt_RefModel/8
  Ground1/1 -> AirPathPlnt_RefModel/9
  ECU_qInjTot_PHY/1 -> AirPathPlnt_RefModel/4
  EnvMdl_tEnv_PHY/1 -> AirPathPlnt_RefModel/2
  AirPathPlnt_RefModel/1 -> hPa_2_Pa/1
  AirPathPlnt_RefModel/3 -> kgph_2_kgpsec/1
  AirPathPlnt_RefModel/5 -> hPa_2_Pa1/1
  AirPathPlnt_RefModel/8 -> hPa_2_Pa2/1
  AirPathPlnt_RefModel/25 -> hPa_2_Pa4/1
  AirPathPlnt_RefModel/28 -> hPa_2_Pa5/1
  Memory/1 -> CmbPlnt_RefModel/8
  Memory1/1 -> CmbPlnt_RefModel/7
  AirPathPlnt_RefModel/27 -> 01_2_%/1
  kgph_2_kgpsec1/1 -> EngMdl_mflExhGas_PHY/1
  AirPathPlnt_RefModel/6 -> EngMdl_tAirClrDs_PHY/1, EngMdl_tTChrgdAir_PHY/1
  kgph_2_kgpsec2/1 -> EngMdl_mflFu_PHY/1
  AirPathPlnt_RefModel/24 -> EngMdl_tTrbDs_PHY/1, EngMdl_tExhT_PHY/1
  Chart/2(fcall_ENGPlntComb()) -> CmbPlnt_RefModel/Trigger
  AirPathPlnt_RefModel/29 -> Scope1/1
  Gain/1 -> EngMdl_ratNO2_PHY/1
  AirPathPlnt_RefModel/7 -> Sum5/1  "mflThr"
  AirPathPlnt_RefModel/20 -> Divide8/2, Sum5/2
  Sum5/1 -> Divide8/1
  Divide8/1 -> 100/1
  SFC_func/1 -> Saturation2/1
  CmbPlnt_RefModel/1 -> Saturation3/1, EngMdl_pwrCrksftPwr_PHY/1  "ENG_pwrCrS_kW"
  AirPathPlnt_RefModel/13 -> Mux1/2, kgph_2_kgpsec2/1  "ENG_mflFuel_mp"
  Mux1/1 -> SFC_func/1
  Saturation2/1 -> EngMdl_sfcBrkSpcFuCns_PHY/1  "ENG_Sfc_gpkWh"
  Saturation3/1 -> Mux1/1
  CmbPlnt_RefModel/5 -> Scope1/2
  CmbPlnt_RefModel/4 -> Scope/2
  CmbPlnt_RefModel/3 -> Gain/1, EngMdl_ratNOx_PHY/1
  CmbPlnt_RefModel/2 -> EngMdl_trqEngTqOut_PHY/1
  AirPathPlnt_RefModel/2 -> EngMdl_tAirFilDs_PHY/1
  AirPathPlnt_RefModel/4 -> Term2/1
  AirPathPlnt_RefModel/10 -> Term3/1
  AirPathPlnt_RefModel/11 -> Term4/1
  AirPathPlnt_RefModel/12 -> Term5/1
  AirPathPlnt_RefModel/14 -> Term6/1
  AirPathPlnt_RefModel/15 -> Term7/1
  AirPathPlnt_RefModel/17 -> Term8/1
  AirPathPlnt_RefModel/18 -> Term9/1
  AirPathPlnt_RefModel/21 -> Term10/1
  iSimnTiStep_C_Comb/1 -> Weighted Sample Time Math1/1
  tiSimnTiStep_C/1 -> Weighted Sample Time Math11/1
  Weighted Sample Time Math11/1 -> Chart/1(numStepENGPlntAirPath)
  Weighted Sample Time Math1/1 -> Chart/2(numStepENGPlntComb)
  Cnv1/1 -> EngMdl_pFuRail_PHY/1

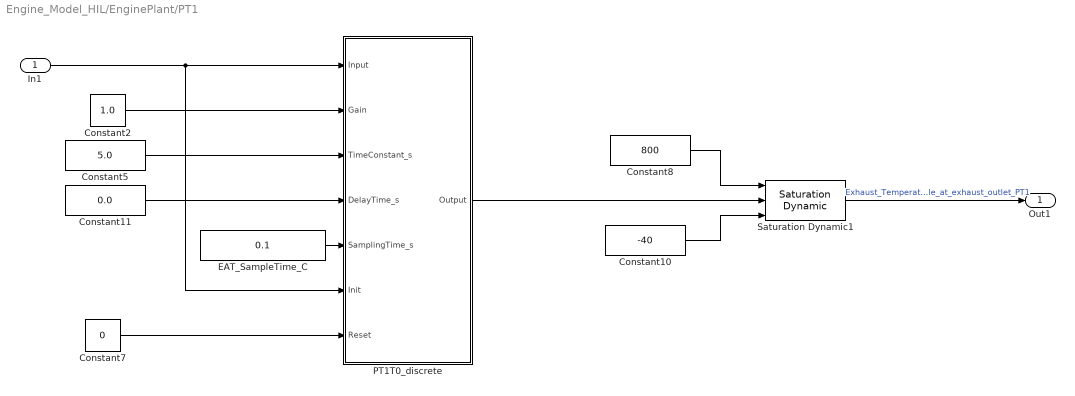
== system Engine_Model_HIL/EnginePlant/PT1 ==
  In1 : Inport
  Constant10 : Constant  Value=-40  OutDataTypeStr=single
  Constant11 : Constant  Value=0.0  OutDataTypeStr=single
  Constant2 : Constant  Value=1.0  OutDataTypeStr=single
  Constant5 : Constant  Value=5.0  OutDataTypeStr=single
  Constant7 : Constant  Value=0  OutDataTypeStr=boolean  SampleTime=-1
  Constant8 : Constant  Value=800  OutDataTypeStr=single
  EAT_SampleTime_C : Constant  Value=0.1
  PT1T0_discrete : Subsystem
  Saturation Dynamic1 : simulink/Discontinuities/Saturation Dynamic  OutMin=[]  OutMax=[]  OutDataTypeStr=Inherit: Same as second input  OutDataType=fixdt(1, 16)  OutScaling=2^-10  DoSatur=off
  Out1 : Outport
  wires:
  Constant10/1 -> Saturation Dynamic1/3
  Saturation Dynamic1/1 -> Out1/1  "Exhaust_Temperature_Thermocouple_at_exhaust_outlet_PT1"
  Constant8/1 -> Saturation Dynamic1/1
  Constant2/1 -> PT1T0_discrete/2(Gain)
  EAT_SampleTime_C/1 -> PT1T0_discrete/5(SamplingTime_s)
  PT1T0_discrete/1(Output) -> Saturation Dynamic1/2
  Constant11/1 -> PT1T0_discrete/4(DelayTime_s)
  Constant7/1 -> PT1T0_discrete/7(Reset)
  Constant5/1 -> PT1T0_discrete/3(TimeConstant_s)
  In1/1 -> PT1T0_discrete/1(Input), PT1T0_discrete/6(Init)

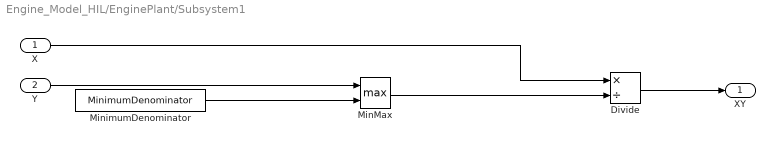
== system Engine_Model_HIL/EnginePlant/Subsystem1 ==
  X : Inport
  Y : Inport  Port=2
  Divide : Product  Inputs=*/  OutDataTypeStr=Inherit: Inherit via back propagation  RndMeth=Nearest  SaturateOnIntegerOverflow=on
      settings: AttributesFormatString=|
      | <OutDT=%<OutDataTypeStr>>
      | <SameDT=%<InputSameDT>>
      | <RndMeth=%<RndMeth>>
      | <SaturateOF=%<SaturateOnIntegerOverflow>>
  MinMax : MinMax  Function=max  Inputs=2  RndMeth=Nearest  ZeroCross=off  InputSameDT=on
      settings: AttributesFormatString=|
      | <OutDT=%<OutDataTypeStr>>
      | <SameDT=%<InputSameDT>>
      | <RndMeth=%<RndMeth>>
      | <SaturateOF=%<SaturateOnIntegerOverflow>>
  MinimumDenominator : Constant  Value=MinimumDenominator  OutDataTypeStr=Inherit: Inherit via back propagation
      settings: AttributesFormatString=<OutDT=%<OutDataTypeStr>>
  XY : Outport
  wires:
  MinMax/1 -> Divide/2
  MinimumDenominator/1 -> MinMax/2
  Y/1 -> MinMax/1
  X/1 -> Divide/1
  Divide/1 -> XY/1

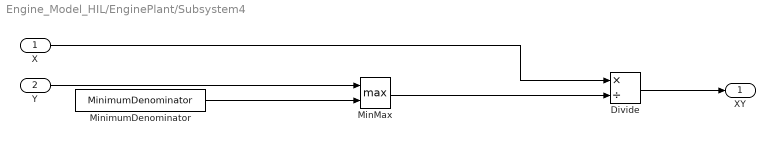
== system Engine_Model_HIL/EnginePlant/Subsystem4 ==
  X : Inport
  Y : Inport  Port=2
  Divide : Product  Inputs=*/  OutDataTypeStr=Inherit: Inherit via back propagation  RndMeth=Nearest  SaturateOnIntegerOverflow=on
      settings: AttributesFormatString=|
      | <OutDT=%<OutDataTypeStr>>
      | <SameDT=%<InputSameDT>>
      | <RndMeth=%<RndMeth>>
      | <SaturateOF=%<SaturateOnIntegerOverflow>>
  MinMax : MinMax  Function=max  Inputs=2  RndMeth=Nearest  ZeroCross=off  InputSameDT=on
      settings: AttributesFormatString=|
      | <OutDT=%<OutDataTypeStr>>
      | <SameDT=%<InputSameDT>>
      | <RndMeth=%<RndMeth>>
      | <SaturateOF=%<SaturateOnIntegerOverflow>>
  MinimumDenominator : Constant  Value=MinimumDenominator  OutDataTypeStr=Inherit: Inherit via back propagation
      settings: AttributesFormatString=<OutDT=%<OutDataTypeStr>>
  XY : Outport
  wires:
  MinMax/1 -> Divide/2
  MinimumDenominator/1 -> MinMax/2
  Y/1 -> MinMax/1
  X/1 -> Divide/1
  Divide/1 -> XY/1

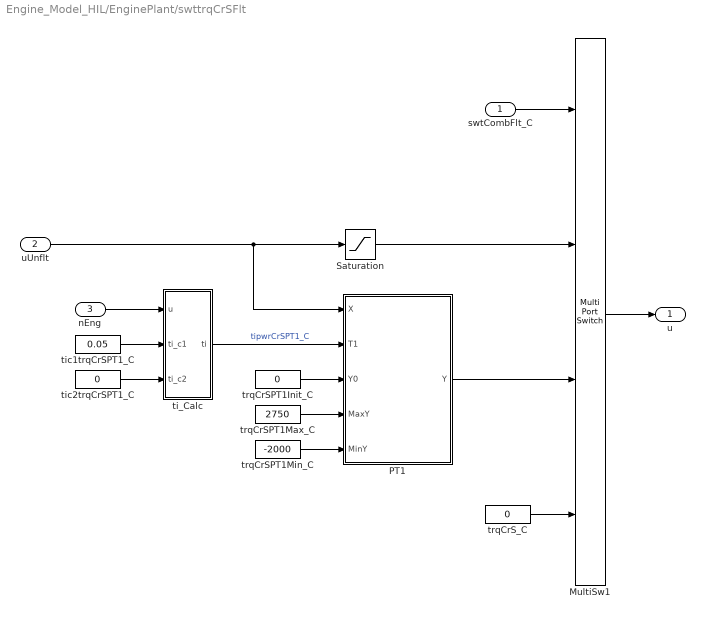
== system Engine_Model_HIL/EnginePlant/swttrqCrSFlt ==
  swtCombFlt_C : Inport
  uUnflt : Inport  Port=2
  nEng : Inport  Port=3
  MultiSw1 : MultiPortSwitch  DataPortOrder=Zero-based contiguous  zeroidx=on
  PT1 : Subsystem
  Saturation : Saturate  UpperLimit=2750  LowerLimit=-2000
  ti_Calc : Subsystem
  tic1trqCrSPT1_C : Constant  Value=0.05  SampleTime=-1
  tic2trqCrSPT1_C : Constant  Value=0  SampleTime=-1
  trqCrSPT1Init_C : Constant  Value=0  SampleTime=-1
  trqCrSPT1Max_C : Constant  Value=2750  SampleTime=-1
  trqCrSPT1Min_C : Constant  Value=-2000  SampleTime=-1
  trqCrS_C : Constant  Value=0  SampleTime=-1
  u : Outport
  wires:
  trqCrS_C/1 -> MultiSw1/4
  uUnflt/1 -> PT1/1(X), Saturation/1
  MultiSw1/1 -> u/1
  nEng/1 -> ti_Calc/1(u)
  tic1trqCrSPT1_C/1 -> ti_Calc/2(ti_c1)
  tic2trqCrSPT1_C/1 -> ti_Calc/3(ti_c2)
  PT1/1(Y) -> MultiSw1/3
  swtCombFlt_C/1 -> MultiSw1/1
  Saturation/1 -> MultiSw1/2
  trqCrSPT1Init_C/1 -> PT1/3(Y0)
  trqCrSPT1Max_C/1 -> PT1/4(MaxY)
  trqCrSPT1Min_C/1 -> PT1/5(MinY)
  ti_Calc/1(ti) -> PT1/2(T1)  "tipwrCrSPT1_C"

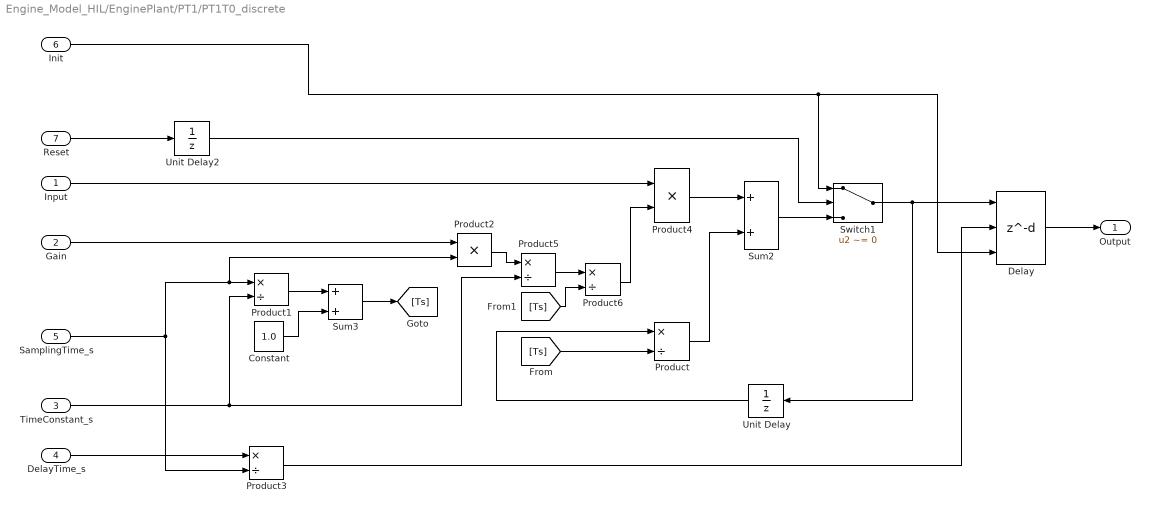
== system Engine_Model_HIL/EnginePlant/PT1/PT1T0_discrete ==
  Input : Inport
  Gain : Inport  Port=2
  TimeConstant_s : Inport  Port=3
  DelayTime_s : Inport  Port=4
  SamplingTime_s : Inport  Port=5
  Init : Inport  Port=6
  Reset : Inport  Port=7
  Constant : Constant  Value=1.0  OutDataTypeStr=single
  Delay : Delay  DelayLengthSource=Input port  InitialConditionSource=Input port
      settings: InputPortMap=u0,p1,p4
  Product{,1,3,5..6} (5 alike) : Product  Inputs=*/  RndMeth=Zero
  Product2 : Product  Inputs=**  RndMeth=Zero
  Product4 : Product  Inputs=**  RndMeth=Zero  OutDataTypeStr=Inherit: Same as first input
  Sum2 : Sum  OutDataTypeStr=Inherit: Same as first input
  Sum3 : Sum
  Switch1 : Switch  Criteria=u2 ~= 0
  Unit Delay : UnitDelay  InitialCondition=0.0  SampleTime=-1
  Unit Delay2 : UnitDelay  InitialCondition=1  SampleTime=-1
  Output : Outport
  wires:
  Input/1 -> Product4/1
  TimeConstant_s/1 -> Product1/2, Product5/2
  Product1/1 -> Sum3/1
  Constant/1 -> Sum3/2
  Sum3/1 -> [Ts]
  [Ts] -> Product/2
  Gain/1 -> Product2/1
  Product5/1 -> Product6/1
  [Ts] -> Product6/2
  Product6/1 -> Product4/2
  Unit Delay/1 -> Product/1
  SamplingTime_s/1 -> Product1/1, Product2/2, Product3/2
  Product2/1 -> Product5/1
  Init/1 -> Switch1/1, Delay/3
  Reset/1 -> Unit Delay2/1
  Product4/1 -> Sum2/1
  Product/1 -> Sum2/2
  Sum2/1 -> Switch1/3
  Switch1/1 -> Unit Delay/1, Delay/1
  Unit Delay2/1 -> Switch1/2
  Delay/1 -> Output/1
  DelayTime_s/1 -> Product3/1
  Product3/1 -> Delay/2

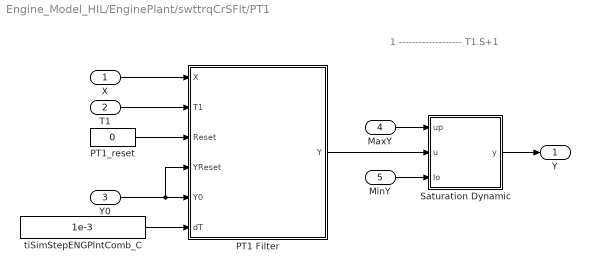
== system Engine_Model_HIL/EnginePlant/swttrqCrSFlt/PT1 ==
  note: 1
      | -------------------
      | T1.S+1
  X : Inport
  T1 : Inport  Port=2
  Y0 : Inport  Port=3
  MaxY : Inport  Port=4
  MinY : Inport  Port=5
  PT1 Filter : Subsystem  mask(PT1 Filter){}
      mask help:
      | Proportional filter with first order time constant, unit gain and external reset.
      |
      | X: Input value
      | T1: Time constant of proportional filter
      | Reset: Reset status
      | YReset: Output value during reset
      | Y0: Initial value of output
      | Y: Output value
      | dT: Sample time
      mask Display:
      | color('blue');
      | fprintf('PT1\nFilter');
      | 
      | color('black');
      | port_label('input', 1, 'X');
      | port_label('input', 2, 'T1');
      | port_label('input', 3, 'Reset');
      | port_label('input', 4, 'YReset');
      | port_label('input', 5, 'Y0');
      | port_label('input', 6, 'dT');
      | port_label('output', 1, 'Y');
  PT1_reset : Constant  Value=0  SampleTime=-1
  Saturation Dynamic : Subsystem  mask(Saturation Dynamic){OutMin=[], OutMax=[], OutDataTypeStr=Inherit: Same as second input, OutputDataTypeScalingMode=Same as second input, OutDataType=fixdt(1, 16), OutScaling=2^-10, LockScale=off, RndMeth=Floor, DoSatur=off}
      mask prompts: OutMin "Simulink:masks:OutputMinimum_MP"; OutMax "Simulink:masks:OutputMaximum_MP"; OutDataTypeStr "Simulink:masks:OutputDataType_MP"; OutputDataTypeScalingMode "Simulink:masks:OutputDataTypeMode_MP"; OutDataType "Simulink:masks:OutputDataTypeegFixdt116Fixdtsingle_MP"; OutScaling "Simulink:masks:OutputScalingSlopeEg29OrSlopeBias_MP"; LockScale "Simulink:masks:LockOutputDataTypeAgainstFxpTools_MP"; RndMeth "Simulink:masks:IntegerRoundingMode_MP"; DoSatur "Simulink:masks:SaturateOnIntegerOverflow_MP"
      mask help: Simulink:masks:SaturationDynamic_MD
      mask init:
      | blkH = gcbh;
      | blkName = getfullname(blkH);
      | 
      | switch_blks = {'Switch','Switch2'}; 
      | for i = 1:length(switch_blks)
      |   set_param([blkName,'/',switch_blks{i}], ...
      |       'RndMeth', RndMeth, ...
      | 	  'DoSatur', DoSatur);
      | end
      | 
      | propBlk = [blkName, '/Data Type Propagation'];
      | 
      | if strcmp(OutputDataTypeScalingMode, 'Same as second input')
      |     set_param(propBlk, 'PropDataTypeMode', 'Inherit via propagation rule', ...
      |                        'PropScalingMode',  'Inherit via propagation rule');
      | else
      |     scaling = OutScaling;
      |     scalingMode = 'Specify via dialog';
      |     switch OutputDataTypeScalingMode
      |       case 'double'
      |         dataType = 'fixdt(''double'')';
      |       case 'single'
      |         dataType = 'fixdt(''single'')';
      |       case 'int8'
      |         dataType = 'fixdt(1,8,0)';
      |       case 'uint8'
      |         dataType = 'fixdt(0,8,0)';
      |       case 'int16'
      |         dataType = 'fixdt(1,16,0)';
      |       case 'uint16'
      |         dataType = 'fixdt(0,16,0)';
      |       case 'int32'
      |         dataType = 'fixdt(1,32,0)';
      |       case 'uint32'
      |         dataType = 'fixdt(0,32,0)';
      |       case 'Specify via dialog'
      |         dataType = OutDataType;
      |         if ~isempty(OutDataTypeStr) && isa(OutDataTypeStr,'Simulink.NumericType') 
      |           if strcmp(OutDataTypeStr.DataTypeMode, 'Fixed-point: unspecified scaling') 
      |             scalingMode = 'Obtain via best precision';
      |             range = [OutMin OutMax];
      |             range = range(~isinf(range));
      |             set_param(propBlk, 'ValuesUsedBestPrec', mat2str(range));
      |           end
      |         end
      |     end
      |     
      |     set_param(propBlk, 'PropDataTypeMode', 'Specify via dialog', ...
      |                        'PropScalingMode',  scalingMode, ...
      |                        'PropDataType',     dataType, ...
      |                        'PropScaling',      scaling);
      | end
      mask Callback OutDataTypeStr: fixptdialog(gcbh)
      mask TypeOptions OutputDataTypeScalingMode: double | single | int8 | uint8 | int16 | uint16 | int32 | uint32 | Specify via dialog | Same as second input
      mask Callback OutputDataTypeScalingMode: fixptdialog(gcbh)
      mask Callback OutDataType: fixptdialog(gcbh)
      mask TypeOptions RndMeth: Simulink:masks:Ceiling | Simulink:masks:Convergent | Simulink:masks:Floor | Simulink:masks:Nearest | Simulink:masks:Round | Simulink:masks:Simplest | Simulink:masks:Zero
      mask Display: plot([0.15 0.85],[.5 .5],[.5 .5],[0.05 0.95],0.15+0.7*[0 .25 .75 1],0.05+0.9*[.25 .25 .75 .75]);
  tiSimStepENGPlntComb_C : Constant  Value=1e-3  SampleTime=-1
  Y : Outport
  wires:
  PT1_reset/1 -> PT1 Filter/3(Reset)
  tiSimStepENGPlntComb_C/1 -> PT1 Filter/6(dT)
  PT1 Filter/1(Y) -> Saturation Dynamic/2(u)
  Saturation Dynamic/1(y) -> Y/1
  Y0/1 -> PT1 Filter/4(YReset), PT1 Filter/5(Y0)
  MinY/1 -> Saturation Dynamic/3(lo)
  X/1 -> PT1 Filter/1(X)
  T1/1 -> PT1 Filter/2(T1)
  MaxY/1 -> Saturation Dynamic/1(up)

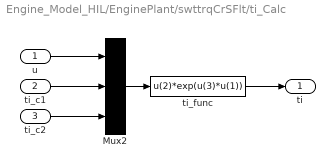
== system Engine_Model_HIL/EnginePlant/swttrqCrSFlt/ti_Calc ==
  u : Inport
  ti_c1 : Inport  Port=2
  ti_c2 : Inport  Port=3
  Mux2 : Mux  Inputs=3
  ti_func : Fcn  Expr=u(2)*exp(u(3)*u(1))
  ti : Outport
  wires:
  ti_c2/1 -> Mux2/3
  ti_c1/1 -> Mux2/2
  ti_func/1 -> ti/1
  Mux2/1 -> ti_func/1
  u/1 -> Mux2/1

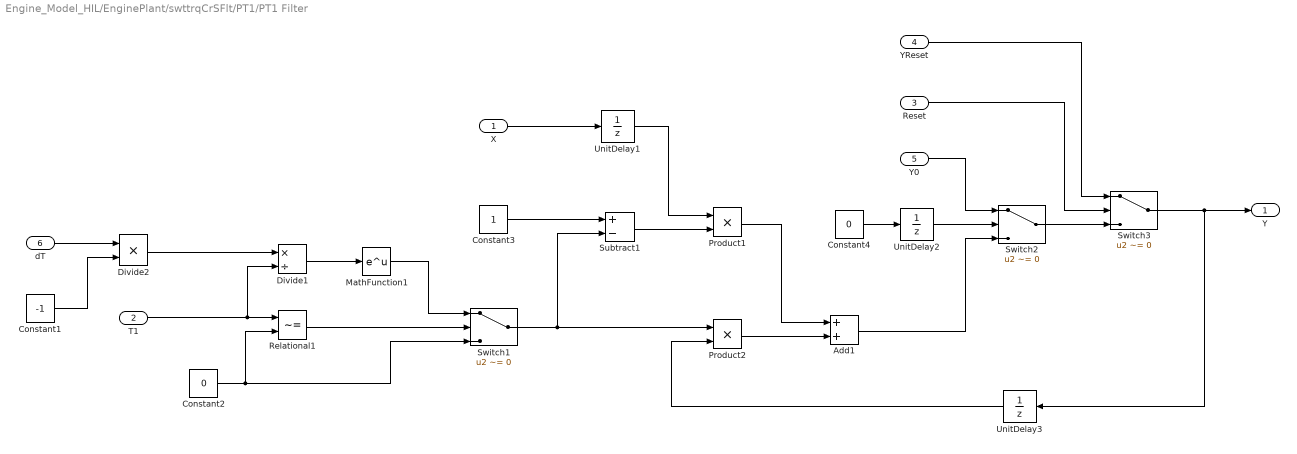
== system Engine_Model_HIL/EnginePlant/swttrqCrSFlt/PT1/PT1 Filter ==
  X : Inport
  T1 : Inport  Port=2
  Reset : Inport  Port=3
  YReset : Inport  Port=4
  Y0 : Inport  Port=5
  dT : Inport  Port=6
  Add1 : Sum
  Constant1 : Constant  Value=-1  SampleTime=-1
  Constant2 : Constant  Value=0  SampleTime=-1
  Constant3 : Constant  SampleTime=-1
  Constant4 : Constant  Value=0  SampleTime=-1
  Divide1 : Product  Inputs=*/
  Divide2 : Product  Inputs=**
  MathFunction1 : Math  SaturateOnIntegerOverflow=on
  Product1 : Product  RndMeth=Zero
  Product2 : Product  RndMeth=Zero
  Relational1 : RelationalOperator  Operator=~=  OutDataTypeStr=boolean  RndMeth=Nearest
  Subtract1 : Sum  Inputs=+-
  Switch1 : Switch  Criteria=u2 ~= 0
  Switch2 : Switch  Criteria=u2 ~= 0
  Switch3 : Switch  Criteria=u2 ~= 0
  UnitDelay1 : UnitDelay  SampleTime=-1
  UnitDelay2 : UnitDelay  InitialCondition=1  SampleTime=-1
  UnitDelay3 : UnitDelay  SampleTime=-1
  Y : Outport
  wires:
  dT/1 -> Divide2/1
  Constant2/1 -> Relational1/2, Switch1/3
  MathFunction1/1 -> Switch1/1
  Relational1/1 -> Switch1/2
  Switch2/1 -> Switch3/3
  Add1/1 -> Switch2/3
  Switch3/1 -> Y/1, UnitDelay3/1
  Y0/1 -> Switch2/1
  UnitDelay2/1 -> Switch2/2
  Constant4/1 -> UnitDelay2/1
  YReset/1 -> Switch3/1
  Reset/1 -> Switch3/2
  UnitDelay3/1 -> Product2/2
  Switch1/1 -> Product2/1, Subtract1/2
  Product2/1 -> Add1/2
  Product1/1 -> Add1/1
  Subtract1/1 -> Product1/2
  UnitDelay1/1 -> Product1/1
  X/1 -> UnitDelay1/1
  Constant3/1 -> Subtract1/1
  Divide1/1 -> MathFunction1/1
  Divide2/1 -> Divide1/1
  T1/1 -> Relational1/1, Divide1/2
  Constant1/1 -> Divide2/2
